simulink model "Plant_0"  (R2024b)
settings: Solver=VariableStepAuto  StartTime=0.0  StopTime=10.0  FixedStep=0.0002  RelTol=1e-3
undefined symbols (not defined in the file or in its folder): g, I1, I2, kd_th1, kd_th2, ki_th1, ki_th2, kp_th1, kp_th2, L1, L2, lc1, lc2, m1, m2, N_th1, N_th2
libraries: simulink x2, slpidlib x2
settings Model: Creator=Sez26  LastModifiedBy=herra

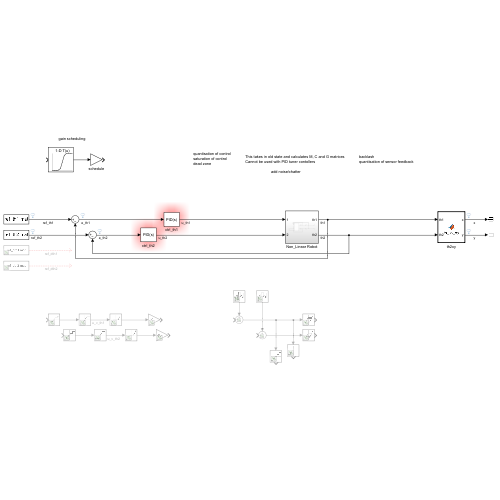
[thumbnail: Simulink's stored preview of the top-level diagram]
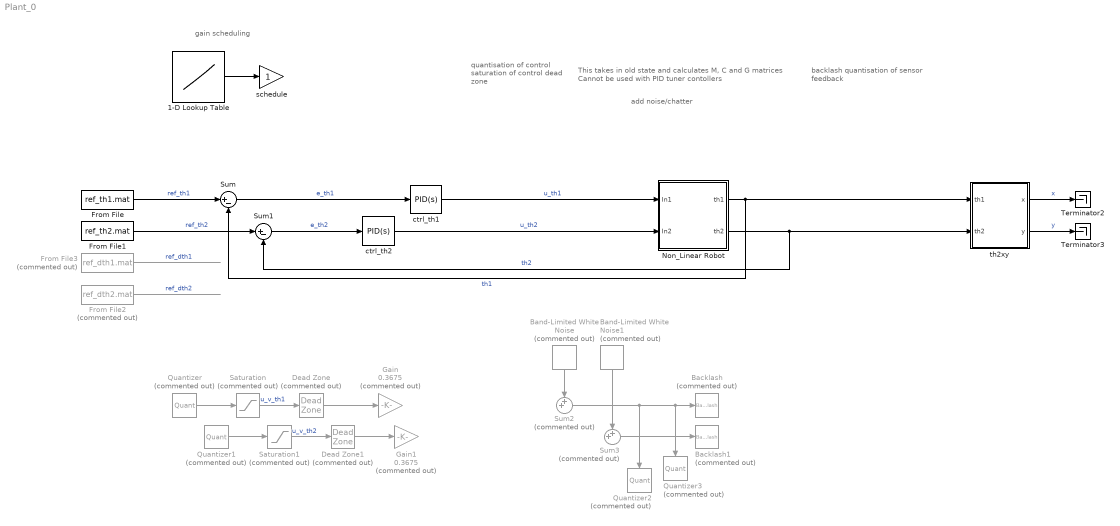
== system Plant_0 ==
  note: gain scheduling
  note: add noise/chatter
  note: backlash
      | quantisation of sensor feedback
  note: quantisation of control
      | saturation of control
      | dead zone
  note: This takes in old state and calculates M, C and G matrices
      | Cannot be used with PID tuner contollers
  1-D Lookup Table : Lookup_n-D  NumberOfTableDimensions=1  BreakpointsForDimension1=[-5:5]  Table=tanh([-5:5])  InternalRulePriority=Speed  RndMeth=Simplest
  Backlash : Backlash  Commented=on  BacklashWidth=2
  Backlash1 : Backlash  Commented=on  BacklashWidth=2
  Band-Limited White Noise : simulink/Sources/Band-Limited White Noise  Commented=on  Cov=[0.17]  Ts=0.02  seed=[23341]
  Band-Limited White Noise1 : simulink/Sources/Band-Limited White Noise  Commented=on  Cov=[0.17]  Ts=0.02  seed=[23341]
  Dead Zone : DeadZone  Commented=on
  Dead Zone1 : DeadZone  Commented=on
  From File : FromFile  FileName=ref_th1.mat  SampleTime=0
  From File1 : FromFile  FileName=ref_th2.mat  SampleTime=0
  From File2 : FromFile  Commented=on  FileName=ref_dth2.mat  SampleTime=0
  From File3 : FromFile  Commented=on  FileName=ref_dth1.mat  SampleTime=0
  Gain : Gain  Commented=on  Gain=0.3675
  Gain1 : Gain  Commented=on  Gain=0.3675
  Non_Linear Robot : Subsystem
  Quantizer : Quantizer  Commented=on  QuantizationInterval=0.05
  Quantizer1 : Quantizer  Commented=on  QuantizationInterval=0.05
  Quantizer2 : Quantizer  Commented=on  QuantizationInterval=0.17
  Quantizer3 : Quantizer  Commented=on  QuantizationInterval=0.17
  Saturation : Saturate  Commented=on  UpperLimit=12  LowerLimit=-12
  Saturation1 : Saturate  Commented=on  UpperLimit=12  LowerLimit=-12
  Sum : Sum  Inputs=|+-
  Sum1 : Sum  Inputs=|+-
  Sum2 : Sum  Commented=on  Inputs=++|
  Sum3 : Sum  Commented=on  Inputs=++|
  Terminator2 : Terminator
  Terminator3 : Terminator
  ctrl_th1 : slpidlib/PID Controller  Controller=PID  Form=Parallel  TimeDomain=Continuous-time  UseExternalTs=off  SampleTime=-1  IntegratorMethod=Forward Euler  FilterMethod=Forward Euler  ControllerParametersSource=internal  P=kp_th1  I=ki_th1  UseKiTs=off  D=kd_th1  UseExternalDerivativeSource=off  N=N_th1  UseFilter=on  TunerSelectOption=Transfer Function Based (PID Tuner App)  InitialConditionSource=internal  InitialConditionForIntegrator=0  InitialConditionForFilter=0  DifferentiatorICPrevScaledInput=0  ExternalReset=none  TrackingMode=off  Kt=1  LimitOutput=off  SatLimitsSource=internal  UpperSaturationLimit=inf  LowerSaturationLimit=-inf  LinearizeAsGain=on  AntiWindupMode=none  Kb=1  LimitIntegrator=off  UpperIntegratorSaturationLimit=inf  LowerIntegratorSaturationLimit=-inf  POutMin=[]  POutMax=[]  IOutMin=[]  IOutMax=[]  DOutMin=[]  DOutMax=[]  NOutMin=[]  NOutMax=[]  SumOutMin=[]  SumOutMax=[]  SaturationOutMin=[]  SaturationOutMax=[]  PParamMin=[]  PParamMax=[]  IParamMin=[]  IParamMax=[]  DParamMin=[]  DParamMax=[]  NParamMin=[]  NParamMax=[]  KbParamMin=[]  KbParamMax=[]  KtParamMin=[]  KtParamMax=[]  KbOutMin=[]  KbOutMax=[]  KtOutMin=[]  KtOutMax=[]  IntegratorOutMin=[]  IntegratorOutMax=[]  FilterOutMin=[]  FilterOutMax=[]  SumI1OutMin=[]  SumI1OutMax=[]  SumI2OutMin=[]  SumI2OutMax=[]  SumI3OutMin=[]  SumI3OutMax=[]  SumI4OutMin=[]  SumI4OutMax=[]  SumDOutMin=[]  SumDOutMax=[]  DifferentiatorOutMin=[]  DifferentiatorOutMax=[]  FilterDiffOutCoefMin=[]  FilterDiffOutCoefMax=[]  ReciprocalOutMin=[]  ReciprocalOutMax=[]  SumDenOutMin=[]  SumDenOutMax=[]  SumNumOutMin=[]  SumNumOutMax=[]  DivideOutMin=[]  DivideOutMax=[]  UdiffTsProdOutMin=[]  UdiffTsProdOutMax=[]  NTsProdOutMin=[]  NTsProdOutMax=[]  UintegralTsProdOutMin=[]  UintegralTsProdOutMax=[]  UngainTsProdOutMin=[]  UngainTsProdOutMax=[]  ClampingZeroOutDataTypeStr=Inherit: Inherit via back propagation  ClampingZeroOutMin=[]  ClampingZeroOutMax=[]  FilterDenConstantOutDataTypeStr=Inherit: Inherit via back propagation  FilterDenConstantOutMin=[]  FilterDenConstantOutMax=[]  PCopyOutDataTypeStr=Inherit: Inherit via back propagation  PCopyOutMin=[]  PCopyOutMax=[]  NCopyOutDataTypeStr=Inherit: Inherit via back propagation  NCopyOutMin=[]  NCopyOutMax=[]  IntegratorContinuousStateAttributes=''  IntegratorStateMustResolveToSignalObject=off  IntegratorRTWStateStorageClass=Auto  FilterContinuousStateAttributes=''  FilterStateMustResolveToSignalObject=off  FilterRTWStateStorageClass=Auto  ParallelPVariant=InternalParameters  IdealPVariant=Disabled  IVariant=InternalParameters  DVariant=InternalParameters  IntegratorVariant=Continuous  SatVariant=Disabled  AWVariant=Passthrough  PCopyVariant=Disabled  TRVariant=Disabled  FdbkBlocksVariant=Forward  IdealPFdbkVariant=Disabled  SatFdbkVariant=Disabled  DerivativeFilterVariant=ContFilter  NVariant=InternalParameters  NCopyVariant=Disabled  FilterICVariant=InternalICsFilter  IntegratorICVariant=InternalICs  ExternalResetVariant=Disabled  TRSumVariant=Passthrough  SumFdbkVariant=Disabled  SumVariant=Sum_PID  TsampFilterVariant=InternalTs  TsampNgainVariant=Passthrough  TsampIntegralVariant=Disabled_SignalSpec  ExternalSaturationOutDataTypeStr=Inherit: Same as second input  DerivativeSourceVariant=ErrorSignal  PreIntVariant=InternalPreInt
  ctrl_th2 : slpidlib/PID Controller  Controller=PID  Form=Parallel  TimeDomain=Continuous-time  UseExternalTs=off  SampleTime=-1  IntegratorMethod=Forward Euler  FilterMethod=Forward Euler  ControllerParametersSource=internal  P=kp_th2  I=ki_th2  UseKiTs=off  D=kd_th2  UseExternalDerivativeSource=off  N=N_th2  UseFilter=on  TunerSelectOption=Transfer Function Based (PID Tuner App)  InitialConditionSource=internal  InitialConditionForIntegrator=0  InitialConditionForFilter=0  DifferentiatorICPrevScaledInput=0  ExternalReset=none  TrackingMode=off  Kt=1  LimitOutput=off  SatLimitsSource=internal  UpperSaturationLimit=inf  LowerSaturationLimit=-inf  LinearizeAsGain=on  AntiWindupMode=none  Kb=1  LimitIntegrator=off  UpperIntegratorSaturationLimit=inf  LowerIntegratorSaturationLimit=-inf  POutMin=[]  POutMax=[]  IOutMin=[]  IOutMax=[]  DOutMin=[]  DOutMax=[]  NOutMin=[]  NOutMax=[]  SumOutMin=[]  SumOutMax=[]  SaturationOutMin=[]  SaturationOutMax=[]  PParamMin=[]  PParamMax=[]  IParamMin=[]  IParamMax=[]  DParamMin=[]  DParamMax=[]  NParamMin=[]  NParamMax=[]  KbParamMin=[]  KbParamMax=[]  KtParamMin=[]  KtParamMax=[]  KbOutMin=[]  KbOutMax=[]  KtOutMin=[]  KtOutMax=[]  IntegratorOutMin=[]  IntegratorOutMax=[]  FilterOutMin=[]  FilterOutMax=[]  SumI1OutMin=[]  SumI1OutMax=[]  SumI2OutMin=[]  SumI2OutMax=[]  SumI3OutMin=[]  SumI3OutMax=[]  SumI4OutMin=[]  SumI4OutMax=[]  SumDOutMin=[]  SumDOutMax=[]  DifferentiatorOutMin=[]  DifferentiatorOutMax=[]  FilterDiffOutCoefMin=[]  FilterDiffOutCoefMax=[]  ReciprocalOutMin=[]  ReciprocalOutMax=[]  SumDenOutMin=[]  SumDenOutMax=[]  SumNumOutMin=[]  SumNumOutMax=[]  DivideOutMin=[]  DivideOutMax=[]  UdiffTsProdOutMin=[]  UdiffTsProdOutMax=[]  NTsProdOutMin=[]  NTsProdOutMax=[]  UintegralTsProdOutMin=[]  UintegralTsProdOutMax=[]  UngainTsProdOutMin=[]  UngainTsProdOutMax=[]  ClampingZeroOutDataTypeStr=Inherit: Inherit via back propagation  ClampingZeroOutMin=[]  ClampingZeroOutMax=[]  FilterDenConstantOutDataTypeStr=Inherit: Inherit via back propagation  FilterDenConstantOutMin=[]  FilterDenConstantOutMax=[]  PCopyOutDataTypeStr=Inherit: Inherit via back propagation  PCopyOutMin=[]  PCopyOutMax=[]  NCopyOutDataTypeStr=Inherit: Inherit via back propagation  NCopyOutMin=[]  NCopyOutMax=[]  IntegratorContinuousStateAttributes=''  IntegratorStateMustResolveToSignalObject=off  IntegratorRTWStateStorageClass=Auto  FilterContinuousStateAttributes=''  FilterStateMustResolveToSignalObject=off  FilterRTWStateStorageClass=Auto  ParallelPVariant=InternalParameters  IdealPVariant=Disabled  IVariant=InternalParameters  DVariant=InternalParameters  IntegratorVariant=Continuous  SatVariant=Disabled  AWVariant=Passthrough  PCopyVariant=Disabled  TRVariant=Disabled  FdbkBlocksVariant=Forward  IdealPFdbkVariant=Disabled  SatFdbkVariant=Disabled  DerivativeFilterVariant=ContFilter  NVariant=InternalParameters  NCopyVariant=Disabled  FilterICVariant=InternalICsFilter  IntegratorICVariant=InternalICs  ExternalResetVariant=Disabled  TRSumVariant=Passthrough  SumFdbkVariant=Disabled  SumVariant=Sum_PID  TsampFilterVariant=InternalTs  TsampNgainVariant=Passthrough  TsampIntegralVariant=Disabled_SignalSpec  ExternalSaturationOutDataTypeStr=Inherit: Same as second input  DerivativeSourceVariant=ErrorSignal  PreIntVariant=InternalPreInt
  schedule : Gain
  th2xy : MATLAB Function  TreatAsAtomicUnit=on
  wires:
  From File1/1 -> Sum1/1  "ref_th2"
  From File2/1 -> ?  "ref_dth2"
  From File/1 -> Sum/1  "ref_th1"
  From File3/1 -> ?  "ref_dth1"
  th2xy/1(x) -> Terminator2/1  "x"
  th2xy/2(y) -> Terminator3/1  "y"
  Quantizer/1 -> Saturation/1
  Quantizer1/1 -> Saturation1/1
  Saturation/1 -> Dead Zone/1  "u_v_th1"
  Saturation1/1 -> Dead Zone1/1  "u_v_th2"
  Sum2/1 -> Quantizer2/1, Backlash/1, Quantizer3/1
  Band-Limited White Noise/1 -> Sum2/1
  Band-Limited White Noise1/1 -> Sum3/1
  Sum3/1 -> Backlash1/1
  Dead Zone/1 -> Gain/1
  Dead Zone1/1 -> Gain1/1
  Non_Linear Robot/1(th1) -> th2xy/1(th1), Sum/2  "th1"
  Non_Linear Robot/2(th2) -> Sum1/2, th2xy/2(th2)  "th2"
  Sum/1 -> ctrl_th1/1  "e_th1"
  Sum1/1 -> ctrl_th2/1  "e_th2"
  ctrl_th1/1 -> Non_Linear Robot/1(In1)  "u_th1"
  ctrl_th2/1 -> Non_Linear Robot/2(In2)  "u_th2"
  1-D Lookup Table/1 -> schedule/1

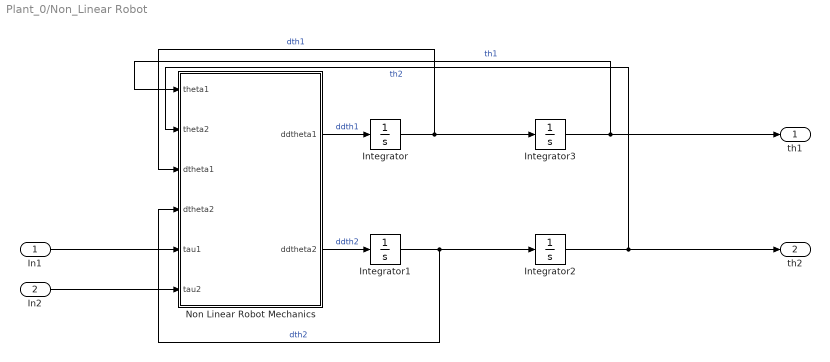
== system Plant_0/Non_Linear Robot ==
  In1 : Inport
  In2 : Inport  Port=2
  Integrator{,1..3} (4 alike) : Integrator
  Non Linear Robot Mechanics : MATLAB Function  TreatAsAtomicUnit=on
  th1 : Outport
  th2 : Outport  Port=2
  wires:
  Integrator1/1 -> Integrator2/1, Non Linear Robot Mechanics/4(dtheta2)  "dth2"
  Integrator2/1 -> th2/1, Non Linear Robot Mechanics/2(theta2)  "th2"
  Integrator3/1 -> th1/1, Non Linear Robot Mechanics/1(theta1)  "th1"
  Non Linear Robot Mechanics/1(ddtheta1) -> Integrator/1  "ddth1"
  In2/1 -> Non Linear Robot Mechanics/6(tau2)
  In1/1 -> Non Linear Robot Mechanics/5(tau1)
  Integrator/1 -> Non Linear Robot Mechanics/3(dtheta1), Integrator3/1  "dth1"
  Non Linear Robot Mechanics/2(ddtheta2) -> Integrator1/1  "ddth2"

== matlab function Plant_0/Non_Linear Robot/Non Linear Robot Mechanics ==
  data: theta1 input; theta2 input; dtheta1 input; dtheta2 input; ddtheta1 output; tau1 input; tau2 input; m2 parameter; m1 parameter; L1 parameter; L2 parameter; I1 parameter; I2 parameter; g parameter; lc1 parameter; lc2 parameter; ddtheta2 output
function [ddtheta1, ddtheta2]= Robot_SS(theta1, theta2, dtheta1, dtheta2, tau1, tau2, m2, m1, L1, L2, I1, I2, g, lc1, lc2)
    % Mass matrix M(theta)
    M11 = m1 * lc1^2 + m2 * (L1^2 + lc2^2 + 2 * L1 * lc2 * cos(theta2)) + I1 + I2;
    M12 = m2 * (lc2^2 + L1 * lc2 * cos(theta2)) + I2;
    M21 = M12;
    M22 = m2 * lc2^2 + I2;
    M = [M11, M12; M21, M22];
    
    % Coriolis matrix C(theta, omega)
    C11 = -m2 * L1 * lc2 * sin(theta2) * dtheta2;
    C12 = -m2 * L1 * lc2 * sin(theta2) * (dtheta1 + dtheta2);
    C21 = m2 * L1 * lc2 * sin(theta2) * dtheta1;
    C22 = 0;
    C = [C11, C12; C21, C22];
    
    % Gravity vector G(theta)
    G1 = (m1 * lc1 + m2 * L1) * g * cos(theta1) + m2 * lc2 * g * cos(theta1 + theta2);
    G2 = m2 * lc2 * g * cos(theta1 + theta2);
    G = [G1; G2];
    
    % Solve for angular accelerations: M * ddtheta = tau - C * dtheta - G
    tau = [tau1; tau2];
    theta_dot = [dtheta1; dtheta2];
    ddtheta = M \ (tau - C * theta_dot - G);
    ddtheta1 = ddtheta(1);
    ddtheta2 = ddtheta(2);

    % calculate new
    % % State-space matrices
    % A = zeros(4, 4);
    % A(1, 3) = 1;
    % A(2, 4) = 1;
    % A(3:4, 3:4) = -M \ C;
    % 
    % B = zeros(4, 2);
    % B(3:4, :) = M \ eye(2);
end

== matlab function Plant_0/th2xy ==
  data: x output; th1 input; y output; th2 input; L1 parameter; L2 parameter
function [x,y] = th_to_xy(th1, th2, L1, L2)
    x = L1*cos(deg2rad(th1)) + L2*cos(deg2rad(th2));
    y = L1*sin(deg2rad(th1)) + L2*sin(deg2rad(th2));
